simulink model "testemplanner_cs"  (R2020a)
settings: Solver=ode5  StartTime=0.0  StopTime=24  FixedStep=1/1000  RelTol=1e-3
PreLoadFcn:
  | mbxruntime.callbacks.PreLoadFcn(bdroot);
PostLoadFcn:
  | mbxruntime.callbacks.PostLoadFcn(bdroot);
InitFcn:
  | mbxruntime.callbacks.InitFcn(bdroot);
StartFcn:
  | mbxruntime.callbacks.StartFcn(bdroot);
StopFcn:
  | mbxruntime.callbacks.StopFcn(bdroot);
model workspace (MAT data in the model file):
  mbox_table : object (value not decoded)
  model_closed = 0
  sim_status = 0
values from neighbouring files (symbols this model uses):
  c_factor = 43.75    [emplanner_init.m]
  cf = -175016    [emplanner_init.m]
  cr = -130634    [emplanner_init.m]
  global_path_x = [0.057304 1.05668625507 2.05480936558 3.05165624935 4.04722112279 5.04150235808 6.03449985569 7.02621407764 8.01664569183 9.00579544113 9.99366409523 10.9802524329 ... (3001 elements, 3001x1)]    [global_path.mat]
  global_path_y = [8.29 8.29 8.29 8.29 8.29 8.29 8.29 8.29 8.29 8.29 8.29 8.29 ... (3001 elements, 3001x1)]    [global_path.mat]
  KD_PID_distance = 0.0    (= 0)    [emplanner_init.m]
  KD_PID_speed = 0    [emplanner_init.m]
  KI_PID_distance = 0.0    (= 0)    [emplanner_init.m]
  KI_PID_speed = 0    [emplanner_init.m]
  KP_PID_distance = 0.5    [emplanner_init.m]
  KP_PID_speed = 1.8    [emplanner_init.m]
  la = 1.265    [emplanner_init.m]
  lb = 2.947-1.265    (= 1.682)    [emplanner_init.m]
  LQR_K1 = k(:,1)'    [emplanner_init.m]
  LQR_K2 = k(:,2)'    [emplanner_init.m]
  LQR_K3 = k(:,3)'    [emplanner_init.m]
  LQR_K4 = k(:,4)'    [emplanner_init.m]
  m = 2020    [emplanner_init.m]
  rack_displacement = [-39.14 , -37.2 , -35.29 , -33.43 , -31.6 , -29.81 , -28.06 , -26.34 , -24.66 ,      -23.01 , -21.38 , -19.79 , -18.23 , -16.69 , -15.18 , -13.7 , -12.23 , -10.8 , -9.38 , -7.98 ,     -6.61 , -5.25 , -3.91 , -2.59 , -1.29 , 0 , 1.27 , 2.54 , 3.78 , 5.02 , 6.24 , 7.46 , 8.66 ,      9.86 , 11.05 , 12.24 , 13.41 , 14.59 , 15.76 , 16.92 , 18.09 , 19.25 , 20.42 , 21.59 , 22.76 ,      23.93 , 25.11 , 26 ...(+26 chars)    [emplanner_init.m]
  right_wheel_ground = [-70 ,-67.2 , -64.4 , -61.6 , -58.8 , -56 , -53.2 , -50.4 , -47.6 , -44.8 , -42 ,      -39.2 , -36.4 , -33.6 , -30.8 , -28 , -25.2 , -22.4 , -19.6 , -16.8 , -14 , -11.2 , -8.4 , -5.6 ,      -2.8 , 0 , 2.8 , 5.6 , 8.4 , 11.2 , 14 , 16.8 , 19.6 , 22.4 , 25.2 , 28 , 30.8 , 33.6 , 36.4 ,      39.2 , 42 , 44.8 , 47.6 , 50.4 , 53.2 , 56 , 58.8 , 61.6 , 64.4 , 67.2 , 70 ]    [emplanner_init.m]
  vx_break_point = zeros(1,5000)    [emplanner_init.m]
undefined symbols (not defined in the file or in its folder): aubr, DiscIntNeverNeededParam, tablebr, vubr
libraries: PreScanSimulinkLibrary x9, Solver_SF x1, simulink_extras x1
(part 4 of 9)

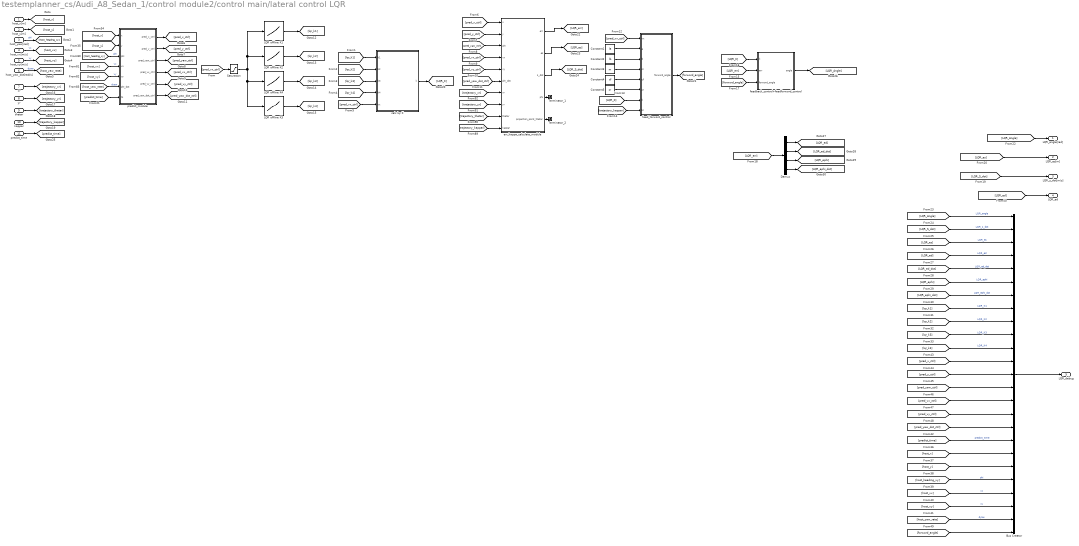
== system testemplanner_cs/Audi_A8_Sedan_1/control module2/control main/lateral control LQR ==
  host_x[m] : Inport
  host_y[m] : Inport  Port=2
  host_yaw[rad] : Inport  Port=3
  host_vx[m/s] : Inport  Port=4
  host_vy[m/s] : Inport  Port=5
  host_yaw_dot[rad/s] : Inport  Port=6
  xr : Inport  Port=7
  yr : Inport  Port=8
  thetar : Inport  Port=9
  kappar : Inport  Port=10
  predict_time : Inport  Port=11
  Bus Creator : BusCreator  Inputs=25
  Constant1 : Constant  Value=la
  Constant2 : Constant  Value=lb
  Constant3 : Constant  Value=m
  Constant4 : Constant  Value=cf
  Constant5 : Constant  Value=cr
  Demux : Demux
  LQR offline K1 : Lookup_n-D  NumberOfTableDimensions=1  BreakpointsForDimension1=vx_break_point  Table=LQR_K1  InternalRulePriority=Speed  RndMeth=Simplest  InputSameDT=on
  LQR offline K2 : Lookup_n-D  NumberOfTableDimensions=1  BreakpointsForDimension1=vx_break_point  Table=LQR_K2  InternalRulePriority=Speed  RndMeth=Simplest  InputSameDT=on
  LQR offline K3 : Lookup_n-D  NumberOfTableDimensions=1  BreakpointsForDimension1=vx_break_point  Table=LQR_K3  InternalRulePriority=Speed  RndMeth=Simplest  InputSameDT=on
  LQR offline K4 : Lookup_n-D  NumberOfTableDimensions=1  BreakpointsForDimension1=vx_break_point  Table=LQR_K4  InternalRulePriority=Speed  RndMeth=Simplest  InputSameDT=on
  Saturation : Saturate  UpperLimit=50  LowerLimit=0
  Terminator_1 : Terminator
  Terminator_2 : Terminator
  calc lqr K : MATLAB Function  TreatAsAtomicUnit=on
  err_kappa_calculate_module : MATLAB Function  TreatAsAtomicUnit=on
  feed_forword_control : MATLAB Function  TreatAsAtomicUnit=on
  feedback_control+feedforword_control : MATLAB Function  TreatAsAtomicUnit=on
  predict_module : MATLAB Function  TreatAsAtomicUnit=on
  LQR_angle[rad] : Outport  VectorParamsAs1DForOutWhenUnconnected=off
  LQR_es[m] : Outport  Port=2  VectorParamsAs1DForOutWhenUnconnected=off
  LQR_s_dot[m/s] : Outport  Port=3  VectorParamsAs1DForOutWhenUnconnected=off
  LQR_ed : Outport  Port=4  VectorParamsAs1DForOutWhenUnconnected=off
  LQR_debug : Outport  Port=5  VectorParamsAs1DForOutWhenUnconnected=off
  wires:
  err_kappa_calculate_module/5(projection_point_thetar) -> Terminator_2/1
  err_kappa_calculate_module/4(phi) -> Terminator_1/1
  [LQR_ed] -> LQR_ed/1
  [forword_angle] -> Bus Creator/25
  [host_yaw_rate] -> Bus Creator/24  "dyaw"
  [host_vy] -> Bus Creator/23  "vy"
  [host_vx] -> Bus Creator/22  "vx"
  [host_heading_xy] -> Bus Creator/21  "phi"
  [host_y] -> Bus Creator/20
  [host_x] -> Bus Creator/19
  [predict_time] -> Bus Creator/18  "predict_time"
  [pred_yaw_dot_ctrl] -> Bus Creator/17
  [pred_vy_ctrl] -> Bus Creator/16
  [pred_vx_ctrl] -> Bus Creator/15
  [pred_yaw_ctrl] -> Bus Creator/14
  [pred_y_ctrl] -> Bus Creator/13
  [pred_x_ctrl] -> Bus Creator/12
  [lqr_k4] -> Bus Creator/11  "LQR_K4"
  [lqr_k3] -> Bus Creator/10  "LQR_K3"
  [lqr_k2] -> Bus Creator/9  "LQR_K2"
  [lqr_k1] -> Bus Creator/8  "LQR_K1"
  [LQR_ephi_dot] -> Bus Creator/7  "LQR_ephi_dot"
  [LQR_ephi] -> Bus Creator/6  "LQR_ephi"
  [LQR_ed_dot] -> Bus Creator/5  "LQR_ed_dot"
  [LQR_ed] -> Bus Creator/4  "LQR_ed"
  Demux/4 -> [LQR_ephi_dot]
  Demux/3 -> [LQR_ephi]
  Demux/2 -> [LQR_ed_dot]
  Demux/1 -> [LQR_ed]
  [LQR_es] -> Bus Creator/3  "LQR_es"
  [LQR_S_dot] -> Bus Creator/2  "LQR_s_dot"
  [LQR_Angle] -> Bus Creator/1  "LQR_angle"
  [LQR_Angle] -> LQR_angle[rad]/1
  feedback_control+feedforword_control/1(angle) -> [LQR_Angle]
  Bus Creator/1 -> LQR_debug/1
  predict_time/1 -> [predict_time]
  Saturation/1 -> LQR offline K1/1, LQR offline K2/1, LQR offline K4/1, LQR offline K3/1
  [LQR_es] -> LQR_es[m]/1
  [LQR_S_dot] -> LQR_s_dot[m/s]/1
  err_kappa_calculate_module/3(s_dot) -> [LQR_S_dot]
  err_kappa_calculate_module/2(es) -> [LQR_es]
  [LQR_err] -> Demux/1
  [forword_angle] -> feedback_control+feedforword_control/3(forword_angle)
  [LQR_K] -> feedback_control+feedforword_control/1(k)
  [LQR_err] -> feedback_control+feedforword_control/2(err)
  err_kappa_calculate_module/1(err) -> [LQR_err]
  feed_forword_control/1(forword_angle) -> [forword_angle]
  [trajectory_kappar] -> feed_forword_control/8(kr)
  [LQR_K] -> feed_forword_control/7(k)
  calc lqr K/1(k) -> [LQR_K]
  Constant5/1 -> feed_forword_control/6(cr)
  Constant4/1 -> feed_forword_control/5(cf)
  Constant3/1 -> feed_forword_control/4(m)
  Constant2/1 -> feed_forword_control/3(b)
  Constant1/1 -> feed_forword_control/2(a)
  [pred_vx_ctrl] -> feed_forword_control/1(vx)
  [trajectory_thetar] -> err_kappa_calculate_module/9(thetar)
  [trajectory_kappar] -> err_kappa_calculate_module/10(kappar)
  [trajectory_yr] -> err_kappa_calculate_module/8(yr)
  [trajectory_xr] -> err_kappa_calculate_module/7(xr)
  kappar/1 -> [trajectory_kappar]
  thetar/1 -> [trajectory_thetar]
  yr/1 -> [trajectory_yr]
  xr/1 -> [trajectory_xr]
  [pred_yaw_dot_ctrl] -> err_kappa_calculate_module/6(phi_dot)
  [pred_vy_ctrl] -> err_kappa_calculate_module/5(vy)
  [pred_vx_ctrl] -> err_kappa_calculate_module/4(vx)
  [pred_yaw_ctrl] -> err_kappa_calculate_module/3("phi ")
  [pred_y_ctrl] -> err_kappa_calculate_module/2(y)
  [pred_x_ctrl] -> err_kappa_calculate_module/1(x)
  [lqr_k1] -> calc lqr K/1(k1)
  [lqr_k2] -> calc lqr K/2(k2)
  [lqr_k3] -> calc lqr K/3(k3)
  [lqr_k4] -> calc lqr K/4(k4)
  [pred_vx_ctrl] -> calc lqr K/5(vx)
  LQR offline K3/1 -> [lqr_k4]
  LQR offline K4/1 -> [lqr_k3]
  LQR offline K2/1 -> [lqr_k2]
  LQR offline K1/1 -> [lqr_k1]
  [pred_vx_ctrl] -> Saturation/1
  predict_module/6(pred_yaw_dot_ctrl) -> [pred_yaw_dot_ctrl]
  predict_module/5(pred_vy_ctrl) -> [pred_vy_ctrl]
  predict_module/4(pred_vx_ctrl) -> [pred_vx_ctrl]
  predict_module/3(pred_yaw_ctrl) -> [pred_yaw_ctrl]
  predict_module/2(pred_y_ctrl) -> [pred_y_ctrl]
  predict_module/1(pred_x_ctrl) -> [pred_x_ctrl]
  host_yaw_dot[rad/s]/1 -> [host_yaw_rate]  "dyaw"
  host_vy[m/s]/1 -> [host_vy]  "vy"
  host_vx[m/s]/1 -> [host_vx]  "vx"
  host_yaw[rad]/1 -> [host_heading_xy]  "phi"
  host_y[m]/1 -> [host_y]
  host_x[m]/1 -> [host_x]
  [predict_time] -> predict_module/7(ts)
  [host_heading_xy] -> predict_module/3(phi)  "phi"
  [host_y] -> predict_module/2(y)
  [host_vx] -> predict_module/4(vx)  "vx"
  [host_yaw_rate] -> predict_module/6(phi_dot)  "dyaw"
  [host_x] -> predict_module/1(x)
  [host_vy] -> predict_module/5(vy)  "vy"

== system testemplanner_cs/Audi_A8_Sedan_1/control module2/control main/longitudinal control double PID ==
  s_err[m] : Inport
  speed_desire[m/s] : Inport  Port=2
  accelerate desire[m/s^2] : Inport  Port=3
  host_speed[m/s] : Inport  Port=4
  host_s_dot[m/s] : Inport  Port=5
  KP_PID_distance : Inport  Port=6
  KI_PID_distance : Inport  Port=7
  KD_PID_distance : Inport  Port=8
  KP_PID_speed : Inport  Port=9
  KI_PID_speed : Inport  Port=10
  KD_PID_speed : Inport  Port=11
  2-D Lookup Table : Lookup_n-D  BreakpointsForDimension1=vubr  BreakpointsForDimension2=aubr  Table=tablebr  InternalRulePriority=Speed  RndMeth=Simplest  InputSameDT=on
  Add : Sum  Inputs=++-
  Add1 : Sum
  Bus Creator : BusCreator  Inputs=9
  Discrete Filter : DiscreteFilter
  MATLAB Function1 : MATLAB Function  TreatAsAtomicUnit=on
  Saturation : Saturate  UpperLimit=45  LowerLimit=-45
  Saturation1 : Saturate  UpperLimit=5  LowerLimit=-8
  discrete pid : Subsystem
  discrete pid1 : Subsystem
  throttle : Outport
  brake : Outport  Port=2
  longitudinal_debug : Outport  Port=3
  wires:
  discrete pid/1(pid_out) -> Add/1
  [KD_PID_speed] -> discrete pid1/4(kd)
  [KI_PID_speed] -> discrete pid1/3(ki)
  [KP_PID_speed] -> discrete pid1/2(kp)
  [KD_PID_distance] -> discrete pid/4(kd)
  [KI_PID_distance] -> discrete pid/3(ki)
  [KP_PID_distance] -> discrete pid/2(kp)
  Discrete Filter/1 -> discrete pid/1(err)
  Bus Creator/1 -> longitudinal_debug/1
  [host_s_dot] -> Bus Creator/9  "host_s_dot"
  [s_err] -> Bus Creator/8  "s_err"
  [host_speed] -> Bus Creator/7  "host_speed"
  [KD_PID_speed] -> Bus Creator/6  "KD_PID_speed"
  [KI_PID_speed] -> Bus Creator/5  "KI_PID_speed"
  [KP_PID_speed] -> Bus Creator/4  "KP_PID_speed"
  [KD_PID_distance] -> Bus Creator/3  "KD_PID_distance"
  [KI_PID_distance] -> Bus Creator/2  "KI_PID_distance"
  [KP_PID_distance] -> Bus Creator/1  "KP_PID_distance"
  MATLAB Function1/2(brake) -> brake/1
  MATLAB Function1/1(throttle) -> throttle/1
  [host_speed] -> 2-D Lookup Table/1
  [host_s_dot] -> Add/3
  host_s_dot[m/s]/1 -> [host_s_dot]
  Saturation1/1 -> 2-D Lookup Table/2
  Add1/1 -> Saturation1/1
  [accelerate_desire] -> Add1/2
  discrete pid1/1(pid_out) -> Add1/1
  Saturation/1 -> discrete pid1/1(err)
  Add/1 -> Saturation/1
  [speed_desire] -> Add/2
  host_speed[m/s]/1 -> [host_speed]
  [s_err] -> Discrete Filter/1
  KD_PID_speed/1 -> [KD_PID_speed]
  KI_PID_speed/1 -> [KI_PID_speed]
  KP_PID_speed/1 -> [KP_PID_speed]
  KD_PID_distance/1 -> [KD_PID_distance]
  KI_PID_distance/1 -> [KI_PID_distance]
  KP_PID_distance/1 -> [KP_PID_distance]
  accelerate desire[m/s^2]/1 -> [accelerate_desire]
  speed_desire[m/s]/1 -> [speed_desire]
  s_err[m]/1 -> [s_err]
  2-D Lookup Table/1 -> MATLAB Function1/1(u)

== system testemplanner_cs/Audi_A8_Sedan_1/control module2/control main/understeer compensate ==
  LQR_angle : Inport
  lateral err : Inport  Port=2
  Add : Sum  Inputs=+-
  Gain : Gain  Gain=0.01
  Manual Switch : ManualSwitch
  LQR_final_angle : Outport
  wires:
  Gain/1 -> Add/2
  LQR_angle/1 -> Manual Switch/1, Add/1
  Manual Switch/1 -> LQR_final_angle/1
  Add/1 -> Manual Switch/2
  lateral err/1 -> Gain/1

== system testemplanner_cs/Audi_A8_Sedan_1/control module3/control main/chassic steering system ==
  LQR_final_angle : Inport
  Constant : Constant  Value=la
  Constant1 : Constant  Value=lb
  Constant17 : Constant  Value=c_factor
  Divide : Product  Inputs=*/
  Gain3 : Gain  Gain=180/pi
  Gain4 : Gain  Gain=360
  MATLAB Function : MATLAB Function  TreatAsAtomicUnit=on
  Saturation : Saturate  UpperLimit=70  LowerLimit=-70
  Saturation1 : Saturate  UpperLimit=1.2217  LowerLimit=-1.2217
  transfer right wheel angle to rack displancement : Lookup_n-D  NumberOfTableDimensions=1  BreakpointsForDimension1=right_wheel_ground  Table=rack_displacement  InternalRulePriority=Speed  RndMeth=Simplest  InputSameDT=on
  lat_steer_sw[deg] : Outport
  wires:
  MATLAB Function/1(right_steer) -> Gain3/1
  Saturation1/1 -> MATLAB Function/1(u)
  LQR_final_angle/1 -> Saturation1/1
  Constant1/1 -> MATLAB Function/3(lb)
  Gain3/1 -> Saturation/1
  Constant/1 -> MATLAB Function/2(la)
  Saturation/1 -> transfer right wheel angle to rack displancement/1
  Divide/1 -> Gain4/1
  Gain4/1 -> lat_steer_sw[deg]/1
  Constant17/1 -> Divide/2
  transfer right wheel angle to rack displancement/1 -> Divide/1

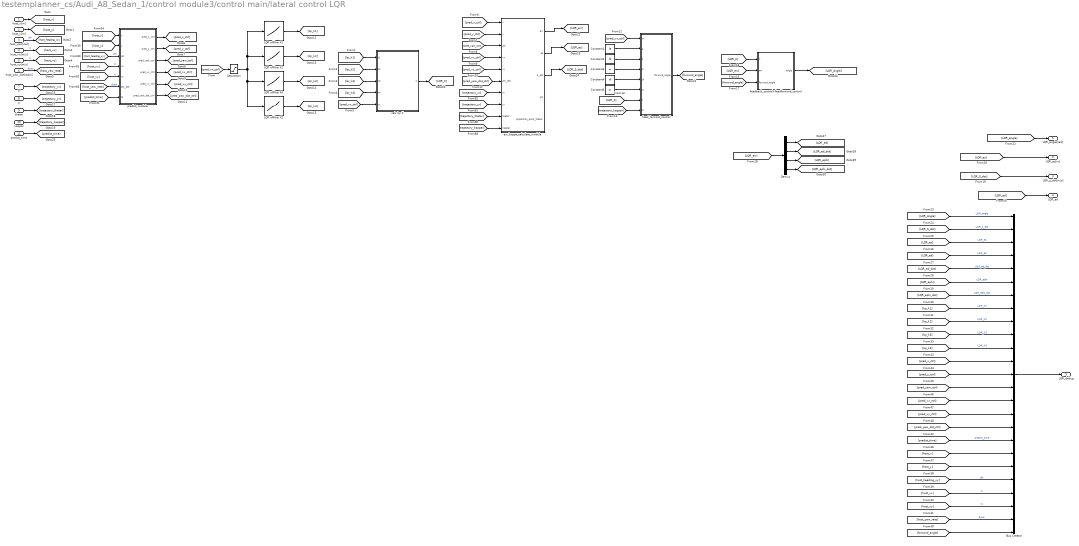
== system testemplanner_cs/Audi_A8_Sedan_1/control module3/control main/lateral control LQR ==
  host_x[m] : Inport
  host_y[m] : Inport  Port=2
  host_yaw[rad] : Inport  Port=3
  host_vx[m/s] : Inport  Port=4
  host_vy[m/s] : Inport  Port=5
  host_yaw_dot[rad/s] : Inport  Port=6
  xr : Inport  Port=7
  yr : Inport  Port=8
  thetar : Inport  Port=9
  kappar : Inport  Port=10
  predict_time : Inport  Port=11
  Bus Creator : BusCreator  Inputs=25
  Constant1 : Constant  Value=la
  Constant2 : Constant  Value=lb
  Constant3 : Constant  Value=m
  Constant4 : Constant  Value=cf
  Constant5 : Constant  Value=cr
  Demux : Demux
  LQR offline K1 : Lookup_n-D  NumberOfTableDimensions=1  BreakpointsForDimension1=vx_break_point  Table=LQR_K1  InternalRulePriority=Speed  RndMeth=Simplest  InputSameDT=on
  LQR offline K2 : Lookup_n-D  NumberOfTableDimensions=1  BreakpointsForDimension1=vx_break_point  Table=LQR_K2  InternalRulePriority=Speed  RndMeth=Simplest  InputSameDT=on
  LQR offline K3 : Lookup_n-D  NumberOfTableDimensions=1  BreakpointsForDimension1=vx_break_point  Table=LQR_K3  InternalRulePriority=Speed  RndMeth=Simplest  InputSameDT=on
  LQR offline K4 : Lookup_n-D  NumberOfTableDimensions=1  BreakpointsForDimension1=vx_break_point  Table=LQR_K4  InternalRulePriority=Speed  RndMeth=Simplest  InputSameDT=on
  Saturation : Saturate  UpperLimit=50  LowerLimit=0
  calc lqr K : MATLAB Function  TreatAsAtomicUnit=on
  err_kappa_calculate_module : MATLAB Function  TreatAsAtomicUnit=on
  feed_forword_control : MATLAB Function  TreatAsAtomicUnit=on
  feedback_control+feedforword_control : MATLAB Function  TreatAsAtomicUnit=on
  predict_module : MATLAB Function  TreatAsAtomicUnit=on
  LQR_angle[rad] : Outport  VectorParamsAs1DForOutWhenUnconnected=off
  LQR_es[m] : Outport  Port=2  VectorParamsAs1DForOutWhenUnconnected=off
  LQR_s_dot[m/s] : Outport  Port=3  VectorParamsAs1DForOutWhenUnconnected=off
  LQR_ed : Outport  Port=4  VectorParamsAs1DForOutWhenUnconnected=off
  LQR_debug : Outport  Port=5  VectorParamsAs1DForOutWhenUnconnected=off
  wires:
  [LQR_ed] -> LQR_ed/1
  [forword_angle] -> Bus Creator/25
  [host_yaw_rate] -> Bus Creator/24  "dyaw"
  [host_vy] -> Bus Creator/23  "vy"
  [host_vx] -> Bus Creator/22  "vx"
  [host_heading_xy] -> Bus Creator/21  "phi"
  [host_y] -> Bus Creator/20
  [host_x] -> Bus Creator/19
  [predict_time] -> Bus Creator/18  "predict_time"
  [pred_yaw_dot_ctrl] -> Bus Creator/17
  [pred_vy_ctrl] -> Bus Creator/16
  [pred_vx_ctrl] -> Bus Creator/15
  [pred_yaw_ctrl] -> Bus Creator/14
  [pred_y_ctrl] -> Bus Creator/13
  [pred_x_ctrl] -> Bus Creator/12
  [lqr_k4] -> Bus Creator/11  "LQR_K4"
  [lqr_k3] -> Bus Creator/10  "LQR_K3"
  [lqr_k2] -> Bus Creator/9  "LQR_K2"
  [lqr_k1] -> Bus Creator/8  "LQR_K1"
  [LQR_ephi_dot] -> Bus Creator/7  "LQR_ephi_dot"
  [LQR_ephi] -> Bus Creator/6  "LQR_ephi"
  [LQR_ed_dot] -> Bus Creator/5  "LQR_ed_dot"
  [LQR_ed] -> Bus Creator/4  "LQR_ed"
  Demux/4 -> [LQR_ephi_dot]
  Demux/3 -> [LQR_ephi]
  Demux/2 -> [LQR_ed_dot]
  Demux/1 -> [LQR_ed]
  [LQR_es] -> Bus Creator/3  "LQR_es"
  [LQR_S_dot] -> Bus Creator/2  "LQR_s_dot"
  [LQR_Angle] -> Bus Creator/1  "LQR_angle"
  [LQR_Angle] -> LQR_angle[rad]/1
  feedback_control+feedforword_control/1(angle) -> [LQR_Angle]
  Bus Creator/1 -> LQR_debug/1
  predict_time/1 -> [predict_time]
  Saturation/1 -> LQR offline K1/1, LQR offline K2/1, LQR offline K4/1, LQR offline K3/1
  [LQR_es] -> LQR_es[m]/1
  [LQR_S_dot] -> LQR_s_dot[m/s]/1
  err_kappa_calculate_module/3(s_dot) -> [LQR_S_dot]
  err_kappa_calculate_module/2(es) -> [LQR_es]
  [LQR_err] -> Demux/1
  [forword_angle] -> feedback_control+feedforword_control/3(forword_angle)
  [LQR_K] -> feedback_control+feedforword_control/1(k)
  [LQR_err] -> feedback_control+feedforword_control/2(err)
  err_kappa_calculate_module/1(err) -> [LQR_err]
  feed_forword_control/1(forword_angle) -> [forword_angle]
  [trajectory_kappar] -> feed_forword_control/8(kr)
  [LQR_K] -> feed_forword_control/7(k)
  calc lqr K/1(k) -> [LQR_K]
  Constant5/1 -> feed_forword_control/6(cr)
  Constant4/1 -> feed_forword_control/5(cf)
  Constant3/1 -> feed_forword_control/4(m)
  Constant2/1 -> feed_forword_control/3(b)
  Constant1/1 -> feed_forword_control/2(a)
  [pred_vx_ctrl] -> feed_forword_control/1(vx)
  [trajectory_thetar] -> err_kappa_calculate_module/9(thetar)
  [trajectory_kappar] -> err_kappa_calculate_module/10(kappar)
  [trajectory_yr] -> err_kappa_calculate_module/8(yr)
  [trajectory_xr] -> err_kappa_calculate_module/7(xr)
  kappar/1 -> [trajectory_kappar]
  thetar/1 -> [trajectory_thetar]
  yr/1 -> [trajectory_yr]
  xr/1 -> [trajectory_xr]
  [pred_yaw_dot_ctrl] -> err_kappa_calculate_module/6(phi_dot)
  [pred_vy_ctrl] -> err_kappa_calculate_module/5(vy)
  [pred_vx_ctrl] -> err_kappa_calculate_module/4(vx)
  [pred_yaw_ctrl] -> err_kappa_calculate_module/3("phi ")
  [pred_y_ctrl] -> err_kappa_calculate_module/2(y)
  [pred_x_ctrl] -> err_kappa_calculate_module/1(x)
  [lqr_k1] -> calc lqr K/1(k1)
  [lqr_k2] -> calc lqr K/2(k2)
  [lqr_k3] -> calc lqr K/3(k3)
  [lqr_k4] -> calc lqr K/4(k4)
  [pred_vx_ctrl] -> calc lqr K/5(vx)
  LQR offline K3/1 -> [lqr_k4]
  LQR offline K4/1 -> [lqr_k3]
  LQR offline K2/1 -> [lqr_k2]
  LQR offline K1/1 -> [lqr_k1]
  [pred_vx_ctrl] -> Saturation/1
  predict_module/6(pred_yaw_dot_ctrl) -> [pred_yaw_dot_ctrl]
  predict_module/5(pred_vy_ctrl) -> [pred_vy_ctrl]
  predict_module/4(pred_vx_ctrl) -> [pred_vx_ctrl]
  predict_module/3(pred_yaw_ctrl) -> [pred_yaw_ctrl]
  predict_module/2(pred_y_ctrl) -> [pred_y_ctrl]
  predict_module/1(pred_x_ctrl) -> [pred_x_ctrl]
  host_yaw_dot[rad/s]/1 -> [host_yaw_rate]  "dyaw"
  host_vy[m/s]/1 -> [host_vy]  "vy"
  host_vx[m/s]/1 -> [host_vx]  "vx"
  host_yaw[rad]/1 -> [host_heading_xy]  "phi"
  host_y[m]/1 -> [host_y]
  host_x[m]/1 -> [host_x]
  [predict_time] -> predict_module/7(ts)
  [host_heading_xy] -> predict_module/3(phi)  "phi"
  [host_y] -> predict_module/2(y)
  [host_vx] -> predict_module/4(vx)  "vx"
  [host_yaw_rate] -> predict_module/6(phi_dot)  "dyaw"
  [host_x] -> predict_module/1(x)
  [host_vy] -> predict_module/5(vy)  "vy"

== system testemplanner_cs/Audi_A8_Sedan_1/control module3/control main/longitudinal control double PID ==
  s_err[m] : Inport
  speed_desire[m/s] : Inport  Port=2
  accelerate desire[m/s^2] : Inport  Port=3
  host_speed[m/s] : Inport  Port=4
  host_s_dot[m/s] : Inport  Port=5
  KP_PID_distance : Inport  Port=6
  KI_PID_distance : Inport  Port=7
  KD_PID_distance : Inport  Port=8
  KP_PID_speed : Inport  Port=9
  KI_PID_speed : Inport  Port=10
  KD_PID_speed : Inport  Port=11
  2-D Lookup Table : Lookup_n-D  BreakpointsForDimension1=vubr  BreakpointsForDimension2=aubr  Table=tablebr  InternalRulePriority=Speed  RndMeth=Simplest  InputSameDT=on
  Add : Sum  Inputs=++-
  Add1 : Sum
  Bus Creator : BusCreator  Inputs=9
  Discrete Filter : DiscreteFilter
  MATLAB Function1 : MATLAB Function  TreatAsAtomicUnit=on
  Saturation : Saturate  UpperLimit=45  LowerLimit=-45
  Saturation1 : Saturate  UpperLimit=5  LowerLimit=-8
  discrete pid : Subsystem
  discrete pid1 : Subsystem
  throttle : Outport
  brake : Outport  Port=2
  longitudinal_debug : Outport  Port=3
  wires:
  discrete pid/1(pid_out) -> Add/1
  [KD_PID_speed] -> discrete pid1/4(kd)
  [KI_PID_speed] -> discrete pid1/3(ki)
  [KP_PID_speed] -> discrete pid1/2(kp)
  [KD_PID_distance] -> discrete pid/4(kd)
  [KI_PID_distance] -> discrete pid/3(ki)
  [KP_PID_distance] -> discrete pid/2(kp)
  Discrete Filter/1 -> discrete pid/1(err)
  Bus Creator/1 -> longitudinal_debug/1
  [host_s_dot] -> Bus Creator/9  "host_s_dot"
  [s_err] -> Bus Creator/8  "s_err"
  [host_speed] -> Bus Creator/7  "host_speed"
  [KD_PID_speed] -> Bus Creator/6  "KD_PID_speed"
  [KI_PID_speed] -> Bus Creator/5  "KI_PID_speed"
  [KP_PID_speed] -> Bus Creator/4  "KP_PID_speed"
  [KD_PID_distance] -> Bus Creator/3  "KD_PID_distance"
  [KI_PID_distance] -> Bus Creator/2  "KI_PID_distance"
  [KP_PID_distance] -> Bus Creator/1  "KP_PID_distance"
  MATLAB Function1/2(brake) -> brake/1
  MATLAB Function1/1(throttle) -> throttle/1
  [host_speed] -> 2-D Lookup Table/1
  [host_s_dot] -> Add/3
  host_s_dot[m/s]/1 -> [host_s_dot]
  Saturation1/1 -> 2-D Lookup Table/2
  Add1/1 -> Saturation1/1
  [accelerate_desire] -> Add1/2
  discrete pid1/1(pid_out) -> Add1/1
  Saturation/1 -> discrete pid1/1(err)
  Add/1 -> Saturation/1
  [speed_desire] -> Add/2
  host_speed[m/s]/1 -> [host_speed]
  [s_err] -> Discrete Filter/1
  KD_PID_speed/1 -> [KD_PID_speed]
  KI_PID_speed/1 -> [KI_PID_speed]
  KP_PID_speed/1 -> [KP_PID_speed]
  KD_PID_distance/1 -> [KD_PID_distance]
  KI_PID_distance/1 -> [KI_PID_distance]
  KP_PID_distance/1 -> [KP_PID_distance]
  accelerate desire[m/s^2]/1 -> [accelerate_desire]
  speed_desire[m/s]/1 -> [speed_desire]
  s_err[m]/1 -> [s_err]
  2-D Lookup Table/1 -> MATLAB Function1/1(u)

== system testemplanner_cs/Audi_A8_Sedan_1/control module3/control main/understeer compensate ==
  LQR_angle : Inport
  lateral err : Inport  Port=2
  Add : Sum  Inputs=+-
  Gain : Gain  Gain=0.01
  Manual Switch : ManualSwitch
  LQR_final_angle : Outport
  wires:
  Gain/1 -> Add/2
  LQR_angle/1 -> Manual Switch/1, Add/1
  Manual Switch/1 -> LQR_final_angle/1
  Add/1 -> Manual Switch/2
  lateral err/1 -> Gain/1

== system testemplanner_cs/Audi_A8_Sedan_1/decision&planning module/EM Planner/Cartesian2Frenet1 ==
  x_set : Inport
  y_set : Inport  Port=2
  vx_set : Inport  Port=3
  vy_set : Inport  Port=4
  ax_set : Inport  Port=5
  ay_set : Inport  Port=6
  frenet_path_x : Inport  Port=7
  frenet_path_y : Inport  Port=8
  proj_match_point_index_set : Inport  Port=9
  proj_x_set : Inport  Port=10
  proj_y_set : Inport  Port=11
  proj_heading_set : Inport  Port=12
  proj_kappa_set : Inport  Port=13
  index2s : Inport  Port=14
  Bus Creator : BusCreator  Inputs=8
  MATLAB Function : MATLAB Function  TreatAsAtomicUnit=on
  MATLAB Function1 : MATLAB Function  TreatAsAtomicUnit=on
  MATLAB Function2 : MATLAB Function  TreatAsAtomicUnit=on
  Cartesian2FrenetOut : Outport
  wires:
  Bus Creator/1 -> Cartesian2FrenetOut/1
  [ddl_set] -> Bus Creator/8  "ddl_set"
  [l_dot2_set] -> Bus Creator/7  "l_dot2_set"
  [s_dot2_set] -> Bus Creator/6  "s_dot2_set"
  [dl_set] -> Bus Creator/5  "dl_set"
  [l_dot_set] -> Bus Creator/4  "l_dot_set"
  [s_dot_set] -> Bus Creator/3  "s_dot_set"
  [l_set] -> Bus Creator/2  "l_set"
  [s_set] -> Bus Creator/1  "s_set"
  MATLAB Function2/3(ddl_set) -> [ddl_set]
  MATLAB Function2/2(l_dot2_set) -> [l_dot2_set]
  MATLAB Function2/1(s_dot2_set) -> [s_dot2_set]
  [dl_set] -> MATLAB Function2/7(dl_set)
  [s_dot_set] -> MATLAB Function2/6(s_dot_set)
  MATLAB Function1/3(dl_set) -> [dl_set]
  MATLAB Function1/2(l_dot_set) -> [l_dot_set]
  MATLAB Function1/1(s_dot_set) -> [s_dot_set]
  [l_set] -> MATLAB Function2/5(l_set)
  [proj_kappa_set] -> MATLAB Function2/4(proj_kappa_set)
  [proj_heading_set] -> MATLAB Function2/3(proj_heading_set)
  [ay_set] -> MATLAB Function2/2(ay_set)
  [ax_set] -> MATLAB Function2/1(ax_set)
  [proj_kappa_set] -> MATLAB Function1/5(proj_kappa_set)
  [proj_heading_set] -> MATLAB Function1/4(proj_heading_set)
  [vy_set] -> MATLAB Function1/3(vy_set)
  [vx_set] -> MATLAB Function1/2(vx_set)
  [l_set] -> MATLAB Function1/1(l_set)
  MATLAB Function/2(l_set) -> [l_set]
  MATLAB Function/1(s_set) -> [s_set]
  [index2s] -> MATLAB Function/9(index2s)
  [proj_heading_set] -> MATLAB Function/7(proj_heading_set)
  [proj_y_set] -> MATLAB Function/6(proj_y_set)
  [proj_match_point_index_set] -> MATLAB Function/8(proj_match_point_index_set)
  [proj_x_set] -> MATLAB Function/5(proj_x_set)
  [frenet_path_y] -> MATLAB Function/4(frenet_path_y)
  [frenet_path_x] -> MATLAB Function/3(frenet_path_x)
  [y_set] -> MATLAB Function/2(y_set)
  [x_set] -> MATLAB Function/1(x_set)
  index2s/1 -> [index2s]
  proj_kappa_set/1 -> [proj_kappa_set]
  proj_heading_set/1 -> [proj_heading_set]
  proj_y_set/1 -> [proj_y_set]
  proj_x_set/1 -> [proj_x_set]
  proj_match_point_index_set/1 -> [proj_match_point_index_set]
  frenet_path_y/1 -> [frenet_path_y]
  frenet_path_x/1 -> [frenet_path_x]
  ay_set/1 -> [ay_set]
  ax_set/1 -> [ax_set]
  vy_set/1 -> [vy_set]
  vx_set/1 -> [vx_set]
  y_set/1 -> [y_set]
  x_set/1 -> [x_set]

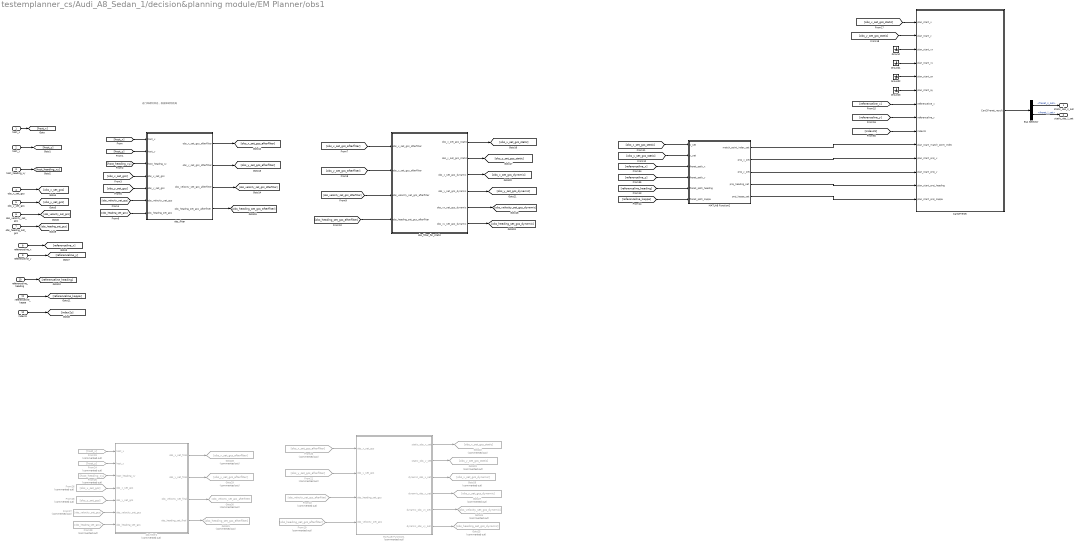
== system testemplanner_cs/Audi_A8_Sedan_1/decision&planning module/EM Planner/obs1 ==
  note: 进行障碍物筛选，根据障碍物距离
  host_x : Inport
  host_y : Inport  Port=2
  host_heading_xy : Inport  Port=3
  obs_x_set_gcs : Inport  Port=4
  obs_y_set_gcs : Inport  Port=5
  obs_velocity_set_gcs : Inport  Port=6
  obs_heading_set_gcs : Inport  Port=7
  referenceline_x : Inport  Port=8
  referenceline_y : Inport  Port=9
  referenceline_heading : Inport  Port=10
  referenceline_kappa : Inport  Port=11
  index2s : Inport  Port=12
  Bus Selector : BusSelector  OutputSignals=frenet_s_set,frenet_l_set
  Cart2Frenet : Subsystem
  From19 : From  Commented=on  GotoTag=obs_heading_set_gcs_afterfliter
  From20 : From  Commented=on  GotoTag=obs_x_set_gcs_afterfliter
  From21 : From  Commented=on  GotoTag=obs_y_set_gcs_afterfliter
  From22 : From  Commented=on  GotoTag=obs_velocity_set_gcs_afterfliter
  From23 : From  Commented=on  GotoTag=host_x
  From24 : From  Commented=on  GotoTag=host_y
  From25 : From  Commented=on  GotoTag=host_heading_xy
  From26 : From  Commented=on  GotoTag=obs_x_set_gcs
  From27 : From  Commented=on  GotoTag=obs_velocity_set_gcs
  From28 : From  Commented=on  GotoTag=obs_y_set_gcs
  From29 : From  Commented=on  GotoTag=obs_heading_set_gcs
  Goto22 : Goto  Commented=on  GotoTag=obs_x_set_gcs_static
  Goto23 : Goto  Commented=on  GotoTag=obs_y_set_gcs_static
  Goto24 : Goto  Commented=on  GotoTag=obs_velocity_set_gcs_dynamic
  Goto25 : Goto  Commented=on  GotoTag=obs_heading_set_gcs_dynamic
  Goto26 : Goto  Commented=on  GotoTag=obs_x_set_gcs_dynamic
  Goto27 : Goto  Commented=on  GotoTag=obs_y_set_gcs_dynamic
  Goto28 : Goto  Commented=on  GotoTag=obs_x_set_gcs_afterfliter
  Goto29 : Goto  Commented=on  GotoTag=obs_y_set_gcs_afterfliter
  Goto30 : Goto  Commented=on  GotoTag=obs_velocity_set_gcs_afterfliter
  Goto31 : Goto  Commented=on  GotoTag=obs_heading_set_gcs_afterfliter
  Ground{,1..3} (4 alike) : Ground
  MATLAB Function1 : MATLAB Function  Commented=on  TreatAsAtomicUnit=on
  MATLAB Function2 : MATLAB Function  TreatAsAtomicUnit=on
  obs filter1 : MATLAB Function  Commented=on  TreatAsAtomicUnit=on
  obs_fliter : MATLAB Function  TreatAsAtomicUnit=on
  obs_fliter_for_static : MATLAB Function  TreatAsAtomicUnit=on
  static_obs_s_set : Outport
  static_obs_l_set : Outport  Port=2
  wires:
  Bus Selector/2 -> static_obs_l_set/1  "<frenet_l_set>"
  Bus Selector/1 -> static_obs_s_set/1  "<frenet_s_set>"
  Cart2Frenet/1(Cart2Frenet_result) -> Bus Selector/1
  MATLAB Function2/5(proj_kappa_set) -> Cart2Frenet/14(plan_start_proj_kappa)
  MATLAB Function2/4(proj_heading_set) -> Cart2Frenet/13(plan_start_proj_heading)
  MATLAB Function2/3(proj_y_set) -> Cart2Frenet/12(plan_start_proj_y)
  MATLAB Function2/2(proj_x_set) -> Cart2Frenet/11(plan_start_proj_x)
  MATLAB Function2/1(match_point_index_set) -> Cart2Frenet/10(plan_start_match_point_index)
  Ground1/1 -> Cart2Frenet/4(plan_start_vy)
  Ground2/1 -> Cart2Frenet/5(plan_start_ax)
  Ground3/1 -> Cart2Frenet/6(plan_start_ay)
  Ground/1 -> Cart2Frenet/3(plan_start_vx)
  [obs_y_set_gcs_static] -> Cart2Frenet/2(plan_start_y)
  [obs_x_set_gcs_static] -> Cart2Frenet/1(plan_start_x)
  [referenceline_y] -> Cart2Frenet/8(referenceline_y)
  [referenceline_x] -> Cart2Frenet/7(referenceline_x)
  [index2s] -> Cart2Frenet/9(index2s)
  [referenceline_kappa] -> MATLAB Function2/6(frenet_path_kappa)
  [referenceline_heading] -> MATLAB Function2/5(frenet_path_heading)
  [referenceline_y] -> MATLAB Function2/4(frenet_path_y)
  [referenceline_x] -> MATLAB Function2/3(frenet_path_x)
  [obs_y_set_gcs_static] -> MATLAB Function2/2(y_set)
  [obs_x_set_gcs_static] -> MATLAB Function2/1(x_set)
  obs_fliter_for_static/6(obs_vy_set_gcs_dynamic) -> [obs_heading_set_gcs_dynamic]
  obs_fliter_for_static/5(obs_vx_set_gcs_dynamic) -> [obs_velocity_set_gcs_dynamic]
  obs_fliter_for_static/4(obs_y_set_gcs_dynamic) -> [obs_y_set_gcs_dynamic]
  obs_fliter_for_static/3(obs_x_set_gcs_dynamic) -> [obs_x_set_gcs_dynamic]
  obs_fliter_for_static/2(obs_y_set_gcs_static) -> [obs_y_set_gcs_static]
  obs_fliter_for_static/1(obs_x_set_gcs_static) -> [obs_x_set_gcs_static]
  [obs_x_set_gcs_afterfliter] -> obs_fliter_for_static/1(obs_x_set_gcs_afterfliter)
  [obs_velocity_set_gcs_afterfliter] -> obs_fliter_for_static/3(obs_velocity_set_gcs_afterfliter)
  [obs_y_set_gcs_afterfliter] -> obs_fliter_for_static/2(obs_y_set_gcs_afterfliter)
  [obs_heading_set_gcs_afterfliter] -> obs_fliter_for_static/4(obs_heading_set_gcs_afterfliter)
  obs_fliter/3(obs_velocity_set_gcs_afterfliter) -> [obs_velocity_set_gcs_afterfliter]
  obs_fliter/4(obs_heading_set_gcs_afterfliter) -> [obs_heading_set_gcs_afterfliter]
  obs_fliter/2(obs_y_set_gcs_afterfliter) -> [obs_y_set_gcs_afterfliter]
  obs_fliter/1(obs_x_set_gcs_afterfliter) -> [obs_x_set_gcs_afterfliter]
  [host_y] -> obs_fliter/2(host_y)
  [host_heading_xy] -> obs_fliter/3(host_heading_xy)
  [obs_x_set_gcs] -> obs_fliter/4(obs_x_set_gcs)
  [obs_y_set_gcs] -> obs_fliter/5(obs_y_set_gcs)
  [obs_velocity_set_gcs] -> obs_fliter/6(obs_velocity_set_gcs)
  [obs_heading_set_gcs] -> obs_fliter/7(obs_heading_set_gcs)
  referenceline_kappa/1 -> [referenceline_kappa]
  referenceline_heading/1 -> [referenceline_heading]
  index2s/1 -> [index2s]
  referenceline_x/1 -> [referenceline_x]
  referenceline_y/1 -> [referenceline_y]
  obs_heading_set_gcs/1 -> [obs_heading_set_gcs]
  obs_velocity_set_gcs/1 -> [obs_velocity_set_gcs]
  obs_y_set_gcs/1 -> [obs_y_set_gcs]
  obs_x_set_gcs/1 -> [obs_x_set_gcs]
  host_heading_xy/1 -> [host_heading_xy]
  host_y/1 -> [host_y]
  host_x/1 -> [host_x]
  [host_x] -> obs_fliter/1(host_x)
  From19/1 -> MATLAB Function1/4(obs_velocity_set_gcs)
  From21/1 -> MATLAB Function1/2(obs_y_set_gcs)
  From22/1 -> MATLAB Function1/3(obs_heading_set_gcs)
  From20/1 -> MATLAB Function1/1(obs_x_set_gcs)
  MATLAB Function1/1(static_obs_x_set) -> Goto22/1
  MATLAB Function1/2(static_obs_y_set) -> Goto23/1
  MATLAB Function1/3(dynamic_obs_x_set) -> Goto26/1
  MATLAB Function1/4(dynamic_obs_y_set) -> Goto27/1
  MATLAB Function1/5(dynamic_obs_vx_set) -> Goto24/1
  MATLAB Function1/6(dynamic_obs_vy_set) -> Goto25/1
  From23/1 -> obs filter1/1(host_x)
  From29/1 -> obs filter1/7(obs_heading_set_gcs)
  From27/1 -> obs filter1/6(obs_velocity_set_gcs)
  From28/1 -> obs filter1/5(obs_y_set_gcs)
  From26/1 -> obs filter1/4(obs_x_set_gcs)
  From25/1 -> obs filter1/3(host_heading_xy)
  From24/1 -> obs filter1/2(host_y)
  obs filter1/1(obs_x_set_final) -> Goto28/1
  obs filter1/2(obs_y_set_final) -> Goto29/1
  obs filter1/4(obs_heading_set_final) -> Goto31/1
  obs filter1/3(obs_velocity_set_final) -> Goto30/1

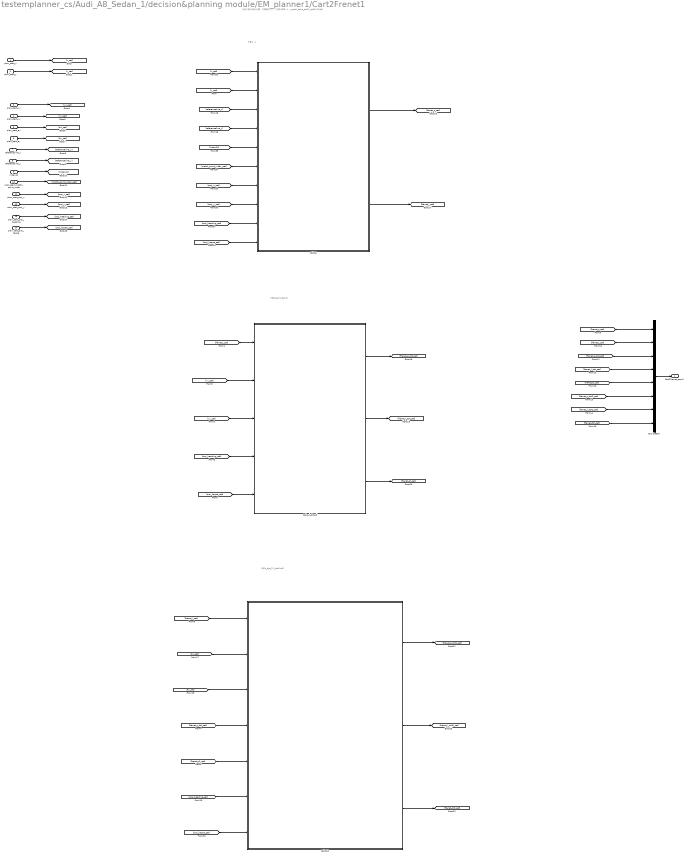
== system testemplanner_cs/Audi_A8_Sedan_1/decision&planning module/EM_planner1/Cart2Frenet1 ==
  note: 分成三部分进行计算，方便后续拆分，分别计算S，L，s_dot,l_dot,s_dot2,l_dot2,dl和ddl
  note: 计算S，L
  note: 计算s_dot,l_dot,dl
  note: 计算s_dot_2,l_dot2,ddl
  plan_start_x : Inport
  plan_start_y : Inport  Port=2
  plan_start_vx : Inport  Port=3
  plan_start_vy : Inport  Port=4
  plan_start_ax : Inport  Port=5
  plan_start_ay : Inport  Port=6
  referenceline_x : Inport  Port=7
  referenceline_y : Inport  Port=8
  index2s : Inport  Port=9
  plan_start_match_point_index : Inport  Port=10
  plan_start_proj_x : Inport  Port=11
  plan_start_proj_y : Inport  Port=12
  plan_start_proj_heading : Inport  Port=13
  plan_start_proj_kappa : Inport  Port=14
  Bus Creator : BusCreator  Inputs=8
  CalcSL : MATLAB Function  TreatAsAtomicUnit=on
  CalcSL2 : MATLAB Function  TreatAsAtomicUnit=on
  Calcs_l_dot_dl : MATLAB Function  TreatAsAtomicUnit=on
  Cart2Frenet_result : Outport
  wires:
  CalcSL/1(frenet_s_set) -> [frenet_s_set]
  plan_start_x/1 -> [x_set]
  plan_start_y/1 -> [y_set]
  plan_start_vx/1 -> [vx_set]
  plan_start_vy/1 -> [vy_set]
  plan_start_ax/1 -> [ax_set]
  plan_start_ay/1 -> [ay_set]
  referenceline_x/1 -> [referenceline_x]
  referenceline_y/1 -> [referenceline_y]
  index2s/1 -> [index2s]
  plan_start_match_point_index/1 -> [match_point_index_set]
  plan_start_proj_x/1 -> [proj_x_set]
  plan_start_proj_y/1 -> [proj_y_set]
  plan_start_proj_heading/1 -> [proj_heading_set]
  plan_start_proj_kappa/1 -> [proj_kappa_set]
  [x_set] -> CalcSL/1(x_set)
  [y_set] -> CalcSL/2(y_set)
  [referenceline_x] -> CalcSL/3(referenceline_x)
  [referenceline_y] -> CalcSL/4(referenceline_y)
  [index2s] -> CalcSL/5(index2s)
  [match_point_index_set] -> CalcSL/6(plan_start_match_point_index)
  [proj_x_set] -> CalcSL/7(plan_start_proj_x)
  [proj_y_set] -> CalcSL/8(plan_start_proj_y)
  [proj_heading_set] -> CalcSL/9(plan_start_proj_heading)
  [proj_kappa_set] -> CalcSL/10(plan_start_proj_kappa)
  [proj_kappa_set] -> Calcs_l_dot_dl/5(plan_start_proj_kappa)
  [proj_heading_set] -> Calcs_l_dot_dl/4(plan_start_proj_heading)
  [vx_set] -> Calcs_l_dot_dl/2(vx_set)
  [proj_heading_set] -> CalcSL2/6(plan_start_proj_heading)
  [proj_kappa_set] -> CalcSL2/7(plan_start_proj_kappa)
  CalcSL/2(frenet_l_set) -> [frenet_l_set]
  [frenet_l_set] -> Calcs_l_dot_dl/1(frenet_l_set)
  [vy_set] -> Calcs_l_dot_dl/3(vy_set)
  Calcs_l_dot_dl/1(s_dot_set) -> [frenet_s_dot_set]
  Calcs_l_dot_dl/2(l_dot_set) -> [frenet_l_dot_set]
  Calcs_l_dot_dl/3(dl_set) -> [frenet_dl_set]
  [ax_set] -> CalcSL2/2(ax_set)
  [ay_set] -> CalcSL2/3(ay_set)
  [frenet_dl_set] -> CalcSL2/5(dl_set)
  [frenet_l_set] -> CalcSL2/1(frenet_l_set)
  [frenet_s_dot_set] -> CalcSL2/4(s_dot_set)
  CalcSL2/3(ddl_set) -> [frenet_ddl_set]
  CalcSL2/2(l_dot2_set) -> [frenet_l_dot2_set]
  CalcSL2/1(s_dot2_set) -> [frenet_s_dot2_set]
  [frenet_s_set] -> Bus Creator/1
  [frenet_l_set] -> Bus Creator/2
  [frenet_s_dot_set] -> Bus Creator/3
  [frenet_l_dot_set] -> Bus Creator/4
  [frenet_dl_set] -> Bus Creator/5
  [frenet_s_dot2_set] -> Bus Creator/6
  [frenet_l_dot2_set] -> Bus Creator/7
  [frenet_ddl_set] -> Bus Creator/8
  Bus Creator/1 -> Cart2Frenet_result/1

== system testemplanner_cs/Audi_A8_Sedan_1/decision&planning module/EM_planner1/Cartesian2Frenet ==
  x_set : Inport
  y_set : Inport  Port=2
  vx_set : Inport  Port=3
  vy_set : Inport  Port=4
  ax_set : Inport  Port=5
  ay_set : Inport  Port=6
  frenet_path_x : Inport  Port=7
  frenet_path_y : Inport  Port=8
  proj_match_point_index_set : Inport  Port=9
  proj_x_set : Inport  Port=10
  proj_y_set : Inport  Port=11
  proj_heading_set : Inport  Port=12
  proj_kappa_set : Inport  Port=13
  index2s : Inport  Port=14
  Bus Creator : BusCreator  Inputs=8
  MATLAB Function : MATLAB Function  TreatAsAtomicUnit=on
  MATLAB Function1 : MATLAB Function  TreatAsAtomicUnit=on
  MATLAB Function2 : MATLAB Function  TreatAsAtomicUnit=on
  Cartesian2FrenetOut : Outport
  wires:
  Bus Creator/1 -> Cartesian2FrenetOut/1
  [ddl_set] -> Bus Creator/8  "ddl_set"
  [l_dot2_set] -> Bus Creator/7  "l_dot2_set"
  [s_dot2_set] -> Bus Creator/6  "s_dot2_set"
  [dl_set] -> Bus Creator/5  "dl_set"
  [l_dot_set] -> Bus Creator/4  "l_dot_set"
  [s_dot_set] -> Bus Creator/3  "s_dot_set"
  [l_set] -> Bus Creator/2  "l_set"
  [s_set] -> Bus Creator/1  "s_set"
  MATLAB Function2/3(ddl_set) -> [ddl_set]
  MATLAB Function2/2(l_dot2_set) -> [l_dot2_set]
  MATLAB Function2/1(s_dot2_set) -> [s_dot2_set]
  [dl_set] -> MATLAB Function2/7(dl_set)
  [s_dot_set] -> MATLAB Function2/6(s_dot_set)
  MATLAB Function1/3(dl_set) -> [dl_set]
  MATLAB Function1/2(l_dot_set) -> [l_dot_set]
  MATLAB Function1/1(s_dot_set) -> [s_dot_set]
  [l_set] -> MATLAB Function2/5(l_set)
  [proj_kappa_set] -> MATLAB Function2/4(proj_kappa_set)
  [proj_heading_set] -> MATLAB Function2/3(proj_heading_set)
  [ay_set] -> MATLAB Function2/2(ay_set)
  [ax_set] -> MATLAB Function2/1(ax_set)
  [proj_kappa_set] -> MATLAB Function1/5(proj_kappa_set)
  [proj_heading_set] -> MATLAB Function1/4(proj_heading_set)
  [vy_set] -> MATLAB Function1/3(vy_set)
  [vx_set] -> MATLAB Function1/2(vx_set)
  [l_set] -> MATLAB Function1/1(l_set)
  MATLAB Function/2(l_set) -> [l_set]
  MATLAB Function/1(s_set) -> [s_set]
  [index2s] -> MATLAB Function/9(index2s)
  [proj_heading_set] -> MATLAB Function/7(proj_heading_set)
  [proj_y_set] -> MATLAB Function/6(proj_y_set)
  [proj_match_point_index_set] -> MATLAB Function/8(proj_match_point_index_set)
  [proj_x_set] -> MATLAB Function/5(proj_x_set)
  [frenet_path_y] -> MATLAB Function/4(frenet_path_y)
  [frenet_path_x] -> MATLAB Function/3(frenet_path_x)
  [y_set] -> MATLAB Function/2(y_set)
  [x_set] -> MATLAB Function/1(x_set)
  index2s/1 -> [index2s]
  proj_kappa_set/1 -> [proj_kappa_set]
  proj_heading_set/1 -> [proj_heading_set]
  proj_y_set/1 -> [proj_y_set]
  proj_x_set/1 -> [proj_x_set]
  proj_match_point_index_set/1 -> [proj_match_point_index_set]
  frenet_path_y/1 -> [frenet_path_y]
  frenet_path_x/1 -> [frenet_path_x]
  ay_set/1 -> [ay_set]
  ax_set/1 -> [ax_set]
  vy_set/1 -> [vy_set]
  vx_set/1 -> [vx_set]
  y_set/1 -> [y_set]
  x_set/1 -> [x_set]

== system testemplanner_cs/Audi_A8_Sedan_1/decision&planning module/EM_planner1/obs ==
  note: 进行障碍物筛选，根据障碍物距离
  host_x : Inport
  host_y : Inport  Port=2
  host_heading_xy : Inport  Port=3
  obs_x_set_gcs : Inport  Port=4
  obs_y_set_gcs : Inport  Port=5
  obs_velocity_set_gcs : Inport  Port=6
  obs_heading_set_gcs : Inport  Port=7
  referenceline_x : Inport  Port=8
  referenceline_y : Inport  Port=9
  referenceline_heading : Inport  Port=10
  referenceline_kappa : Inport  Port=11
  index2s : Inport  Port=12
  Bus Selector : BusSelector  OutputSignals=frenet_s_set,frenet_l_set
  Cart2Frenet : Subsystem
  Ground{,1..3} (4 alike) : Ground
  MATLAB Function2 : MATLAB Function  TreatAsAtomicUnit=on
  obs_fliter : MATLAB Function  TreatAsAtomicUnit=on
  obs_fliter_for_static : MATLAB Function  TreatAsAtomicUnit=on
  static_obs_s_set : Outport
  static_obs_l_set : Outport  Port=2
  wires:
  Bus Selector/2 -> static_obs_l_set/1  "<frenet_l_set>"
  Bus Selector/1 -> static_obs_s_set/1  "<frenet_s_set>"
  Cart2Frenet/1(Cart2Frenet_result) -> Bus Selector/1
  MATLAB Function2/5(proj_kappa_set) -> Cart2Frenet/14(plan_start_proj_kappa)
  MATLAB Function2/4(proj_heading_set) -> Cart2Frenet/13(plan_start_proj_heading)
  MATLAB Function2/3(proj_y_set) -> Cart2Frenet/12(plan_start_proj_y)
  MATLAB Function2/2(proj_x_set) -> Cart2Frenet/11(plan_start_proj_x)
  MATLAB Function2/1(match_point_index_set) -> Cart2Frenet/10(plan_start_match_point_index)
  Ground1/1 -> Cart2Frenet/4(plan_start_vy)
  Ground2/1 -> Cart2Frenet/5(plan_start_ax)
  Ground3/1 -> Cart2Frenet/6(plan_start_ay)
  Ground/1 -> Cart2Frenet/3(plan_start_vx)
  [obs_y_set_gcs_static] -> Cart2Frenet/2(plan_start_y)
  [obs_x_set_gcs_static] -> Cart2Frenet/1(plan_start_x)
  [referenceline_y] -> Cart2Frenet/8(referenceline_y)
  [referenceline_x] -> Cart2Frenet/7(referenceline_x)
  [index2s] -> Cart2Frenet/9(index2s)
  [referenceline_kappa] -> MATLAB Function2/6(frenet_path_kappa)
  [referenceline_heading] -> MATLAB Function2/5(frenet_path_heading)
  [referenceline_y] -> MATLAB Function2/4(frenet_path_y)
  [referenceline_x] -> MATLAB Function2/3(frenet_path_x)
  [obs_y_set_gcs_static] -> MATLAB Function2/2(y_set)
  [obs_x_set_gcs_static] -> MATLAB Function2/1(x_set)
  obs_fliter_for_static/6(obs_heading_set_gcs_dynamic) -> [obs_heading_set_gcs_dynamic]
  obs_fliter_for_static/5(obs_velocity_set_gcs_dynamic) -> [obs_velocity_set_gcs_dynamic]
  obs_fliter_for_static/4(obs_y_set_gcs_dynamic) -> [obs_y_set_gcs_dynamic]
  obs_fliter_for_static/3(obs_x_set_gcs_dynamic) -> [obs_x_set_gcs_dynamic]
  obs_fliter_for_static/2(obs_y_set_gcs_static) -> [obs_y_set_gcs_static]
  obs_fliter_for_static/1(obs_x_set_gcs_static) -> [obs_x_set_gcs_static]
  [obs_x_set_gcs_afterfliter] -> obs_fliter_for_static/1(obs_x_set_gcs_afterfliter)
  [obs_velocity_set_gcs_afterfliter] -> obs_fliter_for_static/3(obs_velocity_set_gcs_afterfliter)
  [obs_y_set_gcs_afterfliter] -> obs_fliter_for_static/2(obs_y_set_gcs_afterfliter)
  [obs_heading_set_gcs_afterfliter] -> obs_fliter_for_static/4(obs_heading_set_gcs_afterfliter)
  obs_fliter/3(obs_velocity_set_gcs_afterfliter) -> [obs_velocity_set_gcs_afterfliter]
  obs_fliter/4(obs_heading_set_gcs_afterfliter) -> [obs_heading_set_gcs_afterfliter]
  obs_fliter/2(obs_y_set_gcs_afterfliter) -> [obs_y_set_gcs_afterfliter]
  obs_fliter/1(obs_x_set_gcs_afterfliter) -> [obs_x_set_gcs_afterfliter]
  [host_y] -> obs_fliter/2(host_y)
  [host_heading_xy] -> obs_fliter/3(host_heading_xy)
  [obs_x_set_gcs] -> obs_fliter/4(obs_x_set_gcs)
  [obs_y_set_gcs] -> obs_fliter/5(obs_y_set_gcs)
  [obs_velocity_set_gcs] -> obs_fliter/6(obs_velocity_set_gcs)
  [obs_heading_set_gcs] -> obs_fliter/7(obs_heading_set_gcs)
  referenceline_kappa/1 -> [referenceline_kappa]
  referenceline_heading/1 -> [referenceline_heading]
  index2s/1 -> [index2s]
  referenceline_x/1 -> [referenceline_x]
  referenceline_y/1 -> [referenceline_y]
  obs_heading_set_gcs/1 -> [obs_heading_set_gcs]
  obs_velocity_set_gcs/1 -> [obs_velocity_set_gcs]
  obs_y_set_gcs/1 -> [obs_y_set_gcs]
  obs_x_set_gcs/1 -> [obs_x_set_gcs]
  host_heading_xy/1 -> [host_heading_xy]
  host_y/1 -> [host_y]
  host_x/1 -> [host_x]
  [host_x] -> obs_fliter/1(host_x)

== system testemplanner_cs/Box_1/SELF_Demux/compas converter/cart2compas ==
  Angle [deg] : Inport
  Constant : Constant  Value=90
  Constant1 : Constant  Value=360
  Gain : Gain  Gain=1/360
  Gain1 : Gain  Gain=360
  Gain2 : Gain  Gain=-1
  Rounding Function : Rounding
  Sum : Sum  Inputs=|-+
  Sum1 : Sum  Inputs=-+|
  Sum2 : Sum  Inputs=++|
  heading [deg] : Outport
  wires:
  Gain/1 -> Rounding Function/1
  Rounding Function/1 -> Gain1/1
  Gain1/1 -> Sum/1
  Angle [deg]/1 -> Sum1/2
  Sum/1 -> Gain2/1
  Sum1/1 -> Gain/1, Sum/2
  Constant/1 -> Sum1/1
  Gain2/1 -> Sum2/2
  Constant1/1 -> Sum2/1
  Sum2/1 -> heading [deg]/1

== system testemplanner_cs/Audi_A8_Sedan_1/Trajectories/Traj2State1/Traj2State2/MuxState ==
  x [m] : Inport
  y [m] : Inport  Port=2
  z [m] : Inport  Port=3
  dx [m/s] : Inport  Port=4
  dy [m/s] : Inport  Port=5
  dz [m/s] : Inport  Port=6
  R [rad] : Inport  Port=7
  P [rad] : Inport  Port=8
  Y [rad] : Inport  Port=9
  Mux : Mux  Inputs=9
  state : Outport
  wires:
  z [m]/1 -> Mux/3
  y [m]/1 -> Mux/2
  x [m]/1 -> Mux/1
  Y [rad]/1 -> Mux/9
  P [rad]/1 -> Mux/8
  R [rad]/1 -> Mux/7
  dz [m/s]/1 -> Mux/6
  dy [m/s]/1 -> Mux/5
  dx [m/s]/1 -> Mux/4
  Mux/1 -> state/1

== system testemplanner_cs/Audi_A8_Sedan_1/Trajectories/Traj2State1/Traj2State2/Traj2MuxState_Ext ==
  Traj : Inport
  Terminator{1..9} (9 alike) : Terminator
  demux : Subsystem
  x [m] : Outport
  y [m] : Outport  Port=2
  z [m] : Outport  Port=3
  dx [m/s] : Outport  Port=4
  dy [m/s] : Outport  Port=5
  dz [m/s] : Outport  Port=6
  R [rad] : Outport  Port=7
  P [rad] : Outport  Port=8
  Y [rad] : Outport  Port=9
  wires:
  demux/9(Y) -> Y [rad]/1
  demux/7(R) -> R [rad]/1
  demux/5(vely) -> dy [m/s]/1
  demux/4(velx) -> dx [m/s]/1
  demux/10(velR) -> Terminator4/1
  demux/11(velP) -> Terminator5/1
  demux/12(velY) -> Terminator1/1
  demux/13(accx) -> Terminator8/1
  demux/14(accy) -> Terminator9/1
  demux/15(accz) -> Terminator7/1
  demux/18(accY) -> Terminator2/1
  demux/16(accR) -> Terminator3/1
  demux/17(accP) -> Terminator6/1
  demux/3(z) -> z [m]/1
  Traj/1 -> demux/1(traj)
  demux/6(velz) -> dz [m/s]/1
  demux/1(x) -> x [m]/1
  demux/2(y) -> y [m]/1
  demux/8(P) -> P [rad]/1

== system testemplanner_cs/Audi_A8_Sedan_1/control module2/control main/longitudinal control double PID/discrete pid ==
  err : Inport
  kp : Inport  Port=2
  ki : Inport  Port=3
  kd : Inport  Port=4
  Add2 : Sum  Inputs=+++
  Add3 : Sum
  Add4 : Sum  Inputs=+-
  Delay3 : Delay  DelayLength=1
  Delay4 : Delay  DelayLength=1
  Divide : Product  Inputs=**
  Divide1 : Product  Inputs=**
  Divide2 : Product  Inputs=**
  Gain : Gain  Gain=0.01
  pid_out : Outport
  wires:
  Gain/1 -> Delay3/1
  kd/1 -> [KD_PID_distance]
  ki/1 -> [KI_PID_distance]
  kp/1 -> [KP_PID_distance]
  Add2/1 -> pid_out/1
  Add4/1 -> Divide2/1
  [KI_PID_distance] -> Divide1/2
  Delay3/1 -> Add3/2
  Divide1/1 -> Add2/2
  [KP_PID_distance] -> Divide/1
  Delay4/1 -> Add4/2
  Add3/1 -> Divide1/1, Gain/1
  Divide2/1 -> Add2/3
  Divide/1 -> Add2/1
  err/1 -> Add4/1, Add3/1, Divide/2, Delay4/1
  [KD_PID_distance] -> Divide2/2

== system testemplanner_cs/Audi_A8_Sedan_1/control module2/control main/longitudinal control double PID/discrete pid1 ==
  err : Inport
  kp : Inport  Port=2
  ki : Inport  Port=3
  kd : Inport  Port=4
  Add2 : Sum  Inputs=+++
  Add3 : Sum
  Add4 : Sum  Inputs=+-
  Delay3 : Delay  DelayLength=1
  Delay4 : Delay  DelayLength=1
  Divide : Product  Inputs=**
  Divide1 : Product  Inputs=**
  Divide2 : Product  Inputs=**
  Gain : Gain  Gain=0.01
  pid_out : Outport
  wires:
  [KD_PID_distance] -> Divide2/2
  err/1 -> Delay4/1, Divide/2, Add3/1, Add4/1
  Divide/1 -> Add2/1
  Divide2/1 -> Add2/3
  Add3/1 -> Gain/1, Divide1/1
  Delay4/1 -> Add4/2
  [KP_PID_distance] -> Divide/1
  Divide1/1 -> Add2/2
  Delay3/1 -> Add3/2
  [KI_PID_distance] -> Divide1/2
  Add4/1 -> Divide2/1
  Add2/1 -> pid_out/1
  kp/1 -> [KP_PID_distance]
  ki/1 -> [KI_PID_distance]
  kd/1 -> [KD_PID_distance]
  Gain/1 -> Delay3/1

== system testemplanner_cs/Audi_A8_Sedan_1/control module3/control main/longitudinal control double PID/discrete pid ==
  err : Inport
  kp : Inport  Port=2
  ki : Inport  Port=3
  kd : Inport  Port=4
  Add2 : Sum  Inputs=+++
  Add3 : Sum
  Add4 : Sum  Inputs=+-
  Delay3 : Delay  DelayLength=1
  Delay4 : Delay  DelayLength=1
  Divide : Product  Inputs=**
  Divide1 : Product  Inputs=**
  Divide2 : Product  Inputs=**
  Gain : Gain  Gain=0.01
  pid_out : Outport
  wires:
  Gain/1 -> Delay3/1
  kd/1 -> [KD_PID_distance]
  ki/1 -> [KI_PID_distance]
  kp/1 -> [KP_PID_distance]
  Add2/1 -> pid_out/1
  Add4/1 -> Divide2/1
  [KI_PID_distance] -> Divide1/2
  Delay3/1 -> Add3/2
  Divide1/1 -> Add2/2
  [KP_PID_distance] -> Divide/1
  Delay4/1 -> Add4/2
  Add3/1 -> Divide1/1, Gain/1
  Divide2/1 -> Add2/3
  Divide/1 -> Add2/1
  err/1 -> Add4/1, Add3/1, Divide/2, Delay4/1
  [KD_PID_distance] -> Divide2/2

== system testemplanner_cs/Audi_A8_Sedan_1/control module3/control main/longitudinal control double PID/discrete pid1 ==
  err : Inport
  kp : Inport  Port=2
  ki : Inport  Port=3
  kd : Inport  Port=4
  Add2 : Sum  Inputs=+++
  Add3 : Sum
  Add4 : Sum  Inputs=+-
  Delay3 : Delay  DelayLength=1
  Delay4 : Delay  DelayLength=1
  Divide : Product  Inputs=**
  Divide1 : Product  Inputs=**
  Divide2 : Product  Inputs=**
  Gain : Gain  Gain=0.01
  pid_out : Outport
  wires:
  [KD_PID_distance] -> Divide2/2
  err/1 -> Delay4/1, Divide/2, Add3/1, Add4/1
  Divide/1 -> Add2/1
  Divide2/1 -> Add2/3
  Add3/1 -> Gain/1, Divide1/1
  Delay4/1 -> Add4/2
  [KP_PID_distance] -> Divide/1
  Divide1/1 -> Add2/2
  Delay3/1 -> Add3/2
  [KI_PID_distance] -> Divide1/2
  Add4/1 -> Divide2/1
  Add2/1 -> pid_out/1
  kp/1 -> [KP_PID_distance]
  ki/1 -> [KI_PID_distance]
  kd/1 -> [KD_PID_distance]
  Gain/1 -> Delay3/1
